simulink model "Q1_c"  (R2020b)
settings: Solver=VariableStepAuto  StartTime=0.0  StopTime=60.0  RelTol=1e-3
settings Model: Creator=aloks  LastModifiedBy=aloks

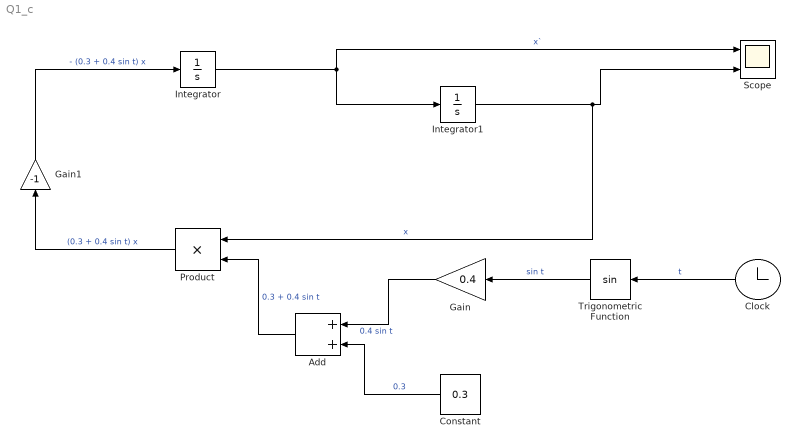
== system Q1_c ==
  Add : Sum
  Clock : Clock
  Constant : Constant  Value=0.3
  Gain : Gain  Gain=0.4
  Gain1 : Gain  Gain=-1
  Integrator : Integrator  InitialCondition=0.2
  Integrator1 : Integrator  InitialCondition=1
  Product : Product
  Scope : Scope  NumInputPorts=2
  Trigonometric Function : Trigonometry
  wires:
  Integrator/1 -> Integrator1/1, Scope/1  "x`"
  Integrator1/1 -> Product/1, Scope/2  "x"
  Clock/1 -> Trigonometric Function/1  "t"
  Trigonometric Function/1 -> Gain/1  "sin t"
  Gain/1 -> Add/1  "0.4 sin t"
  Constant/1 -> Add/2  "0.3"
  Add/1 -> Product/2  "0.3 + 0.4 sin t"
  Product/1 -> Gain1/1  "(0.3 + 0.4 sin t) x"
  Gain1/1 -> Integrator/1  "- (0.3 + 0.4 sin t) x"
